simulink model "valutazione_K_cr"  (R2021b)
settings: Solver=FixedStepAuto  StartTime=0.0  StopTime=50  FixedStep=0.01  RelTol=1e-3
values from neighbouring files (symbols this model uses):
  Kcr = 0.480    (= 0.48)    [script.m]
  r = 1    [script.m]
libraries: cstblocks x1
settings Model: Creator=antony  LastModifiedBy=antony

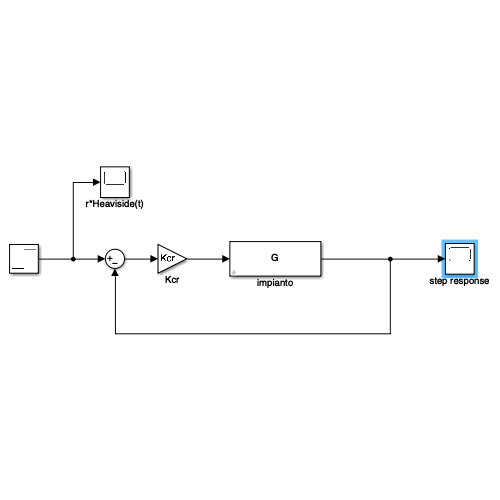
[thumbnail: Simulink's stored preview of the top-level diagram]
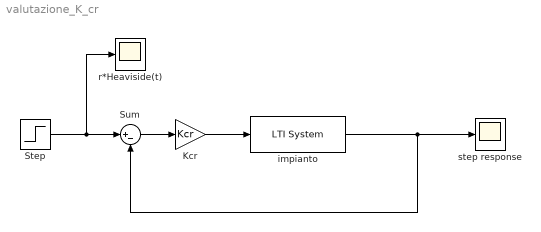
== system valutazione_K_cr ==
  Kcr : Gain  Gain=Kcr
  Step : Step  Time=0  After=r  SampleTime=0
  Sum : Sum  Inputs=|+-
  impianto : cstblocks/LTI System  sys=G  IC=[]
  r*Heaviside(t) : Scope
  step response : Scope
  wires:
  Kcr/1 -> impianto/1
  Step/1 -> Sum/1, r*Heaviside(t)/1
  impianto/1 -> Sum/2, step response/1
  Sum/1 -> Kcr/1
